simulink model "compressor"  (Simulink 7.4)
settings: Solver=ode45  StartTime=0.0  StopTime=10  MaxStep=0.01  RelTol=1e-3
values from neighbouring files (symbols this model uses):
  D = [-0.0083454 -0.0094965 0.16826 -0.032215 -0.61199 0.94175 -0.48522 0.10369]    [comp_coeffs.m]
  x_init_lin = [0.898 ... (first row only)    [MpcSetup.m]    (also in MpcSetup_linearized.m; compressor_setup.m; setup_compressor.m; test2.m = [0.899; 1.125; 0.1512; 440.7; 0])
libraries: dspsrcs4 x2, dspsnks4 x2
settings Model: Creator=chkajon  LastModifiedBy=chkajon

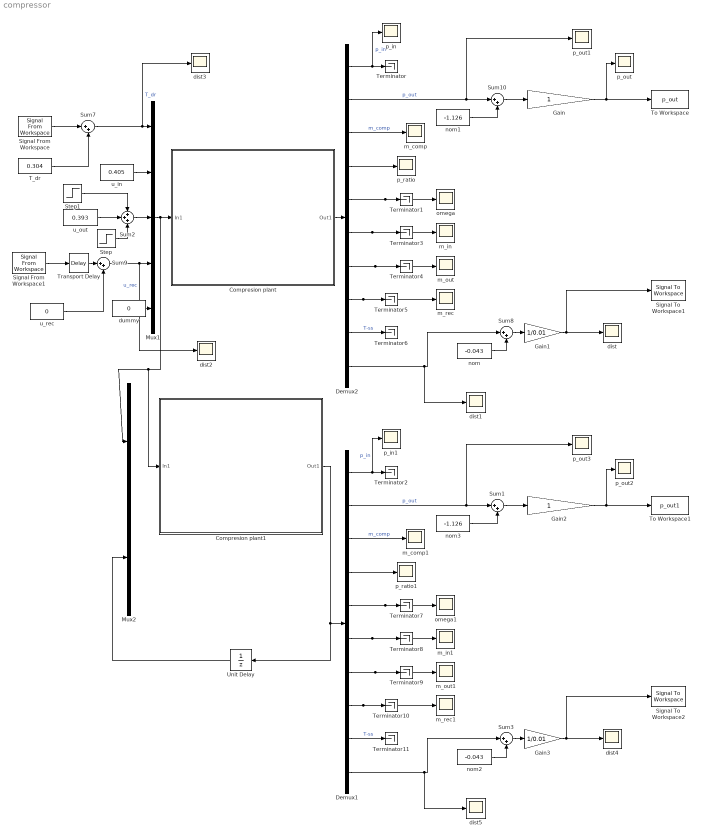
== system compressor ==
  Compresion plant : Subsystem
      mask Display: image(imread('comp_plant.jpg'))
  Compresion plant1 : Subsystem
      mask Display: image(imread('comp_plant.jpg'))
  Demux1 : Demux  Outputs=10
  Demux2 : Demux  Outputs=10
  Gain : Gain
  Gain1 : Gain  Gain=1/0.01
  Gain2 : Gain
  Gain3 : Gain  Gain=1/0.01
  Mux1 : Mux  Inputs=5
  Mux2 : Mux  Inputs=2
  Signal From Workspace : dspsrcs4/Signal From Workspace  SystemSampleTime=-1  X=Td  Ts=1  nsamps=1  OutputAfterFinalValue=Holding final value  ignoreOrWarnInputAndFrameLengths=off
  Signal From Workspace1 : dspsrcs4/Signal From Workspace  SystemSampleTime=-1  X=rec_open  Ts=1  nsamps=1  OutputAfterFinalValue=Holding final value  ignoreOrWarnInputAndFrameLengths=off
  Signal To Workspace1 : dspsnks4/Signal To Workspace  SystemSampleTime=-1  VariableName=SD  FrameMode=Concatenate frames (2-D array)
      settings: FixptAsFi=off
  Signal To Workspace2 : dspsnks4/Signal To Workspace  SystemSampleTime=-1  VariableName=SD1  FrameMode=Concatenate frames (2-D array)
      settings: FixptAsFi=off
  Step : Step  Time=50  After=-0.1  SampleTime=0
  Step1 : Step  Time=100  After=0  SampleTime=0
  Sum{1,3,7..10} (6 alike) : Sum  Inputs=|++
  Sum2 : Sum  Inputs=+++
  T_dr : Constant  Value=0.304
  Terminator{,1..11} (12 alike) : Terminator
  To Workspace : ToWorkspace  VariableName=p_out  SampleTime=-1  SaveFormat=Structure With Time
  To Workspace1 : ToWorkspace  VariableName=p_out1  SampleTime=-1  SaveFormat=Structure With Time
  Transport Delay : TransportDelay  DelayTime=1.0
  Unit Delay : UnitDelay  SampleTime=-1
  dist{,1..5} (6 alike) : Scope
      dist settings: YMin=-11  YMax=2
      dist1 settings: TimeRange=100  YMin=0.03  YMax=0.075
      dist2 settings: TimeRange=100  YMin=-0.25  YMax=1  SaveName=ScopeData3
      dist3 settings: TimeRange=100  YMin=-9  YMax=1  SaveName=ScopeData2
      dist4 settings: YMin=-11  YMax=2  SaveName=ScopeData11
      dist5 settings: TimeRange=100  YMin=0.03  YMax=0.075  SaveName=ScopeData12
  dummy : Constant  Value=0
  m_comp : Scope
      settings: TimeRange=100  YMin=0.5  YMax=0.825  SaveName=m_comp  DataFormat=Array
  m_comp1 : Scope
      settings: TimeRange=100  YMin=0.5  YMax=0.825  SaveName=m_comp1  DataFormat=Array
  m_in : Scope
      settings: TimeRange=100  YMin=100.8  YMax=100.975  SaveName=ScopeData4
  m_in1 : Scope
      settings: TimeRange=100  YMin=100.8  YMax=100.975  SaveName=ScopeData13
  m_out : Scope
      settings: TimeRange=100  YMin=100.8  YMax=100.975  SaveName=ScopeData5
  m_out1 : Scope
      settings: TimeRange=100  YMin=100.8  YMax=100.975  SaveName=ScopeData14
  m_rec : Scope
      settings: TimeRange=100  YMin=100.8  YMax=100.975  SaveName=ScopeData6
  m_rec1 : Scope
      settings: TimeRange=100  YMin=100.8  YMax=100.975  SaveName=ScopeData15
  nom : Constant  Value=-0.043
  nom1 : Constant  Value=-1.126
  nom2 : Constant  Value=-0.043
  nom3 : Constant  Value=-1.126
  omega : Scope
      settings: TimeRange=100  YMin=200  YMax=700  SaveName=ScopeData10
  omega1 : Scope
      settings: TimeRange=100  YMin=200  YMax=700  SaveName=ScopeData16
  p_in : Scope
      settings: TimeRange=100  YMin=0.895197  YMax=0.895225  SaveName=ScopeData9
  p_in1 : Scope
      settings: TimeRange=100  YMin=0.895197  YMax=0.895225  SaveName=ScopeData17
  p_out{,1..3} (4 alike) : Scope
      p_out settings: TimeRange=100  YMin=-2.5  YMax=40  SaveName=ScopeData7
      p_out1 settings: TimeRange=100  YMin=100.8  YMax=100.975  SaveName=ScopeData8
      p_out2 settings: TimeRange=100  YMin=-2.5  YMax=40  SaveName=ScopeData18
      p_out3 settings: TimeRange=100  YMin=100.8  YMax=100.975  SaveName=ScopeData19
  p_ratio : Scope
      settings: TimeRange=100  YMin=0.5  YMax=0.825  SaveName=p_ratio  DataFormat=Array
  p_ratio1 : Scope
      settings: TimeRange=100  YMin=0.5  YMax=0.825  SaveName=p_ratio1  DataFormat=Array
  u_in : Constant  Value=0.405
  u_out : Constant  Value=0.393
  u_rec : Constant  Value=0
  wires:
  Demux2/9 -> Terminator6/1  "T-ss"
  Sum2/1 -> Mux1/3
  Step/1 -> Sum2/3
  Transport Delay/1 -> Sum9/1
  dummy/1 -> Mux1/5
  Demux2/10 -> dist1/1, Sum8/1
  Gain1/1 -> dist/1, Signal To Workspace1/1
  Signal From Workspace/1 -> Sum7/1
  u_rec/1 -> Sum9/2
  T_dr/1 -> Sum7/2
  Gain/1 -> p_out/1, To Workspace/1
  nom1/1 -> Sum10/2
  Sum10/1 -> Gain/1
  Demux2/4 -> p_ratio/1
  Demux2/5 -> omega/1, Terminator1/1
  Demux2/1 -> p_in/1, Terminator/1  "p_in"
  Demux2/2 -> p_out1/1, Sum10/1  "p_out"
  Sum8/1 -> Gain1/1
  nom/1 -> Sum8/2
  Sum9/1 -> dist2/1, Mux1/4  "u_rec"
  Sum7/1 -> Mux1/1, dist3/1  "T_dr"
  Signal From Workspace1/1 -> Transport Delay/1
  u_out/1 -> Sum2/2
  Demux2/7 -> m_out/1, Terminator4/1
  Demux2/8 -> m_rec/1, Terminator5/1
  Demux2/6 -> m_in/1, Terminator3/1
  u_in/1 -> Mux1/2
  Demux2/3 -> m_comp/1  "m_comp"
  Mux1/1 -> Compresion plant/1(In1), Mux2/1, Compresion plant1/1(In1)
  Compresion plant/1(Out1) -> Demux2/1
  Step1/1 -> Sum2/1
  Demux1/9 -> Terminator11/1  "T-ss"
  Demux1/10 -> dist5/1, Sum3/1
  Gain3/1 -> dist4/1, Signal To Workspace2/1
  Gain2/1 -> p_out2/1, To Workspace1/1
  nom3/1 -> Sum1/2
  Sum1/1 -> Gain2/1
  Demux1/4 -> p_ratio1/1
  Demux1/5 -> omega1/1, Terminator7/1
  Demux1/1 -> p_in1/1, Terminator2/1  "p_in"
  Demux1/2 -> p_out3/1, Sum1/1  "p_out"
  Sum3/1 -> Gain3/1
  nom2/1 -> Sum3/2
  Demux1/7 -> m_out1/1, Terminator9/1
  Demux1/8 -> m_rec1/1, Terminator10/1
  Demux1/6 -> m_in1/1, Terminator8/1
  Demux1/3 -> m_comp1/1  "m_comp"
  Compresion plant1/1(Out1) -> Demux1/1, Unit Delay/1
  Unit Delay/1 -> Mux2/2

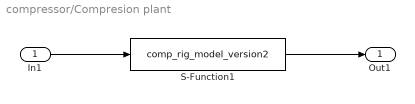
== system compressor/Compresion plant ==
  In1 : Inport
  S-Function1 : S-Function  FunctionName=comp_rig_model_version2  Parameters=[], x_init_lin  EnableBusSupport=off
  Out1 : Outport
  wires:
  In1/1 -> S-Function1/1
  S-Function1/1 -> Out1/1

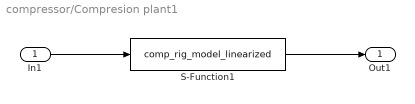
== system compressor/Compresion plant1 ==
  In1 : Inport
  S-Function1 : S-Function  FunctionName=comp_rig_model_linearized  Parameters=[], x_init_lin  EnableBusSupport=off
  Out1 : Outport
  wires:
  In1/1 -> S-Function1/1
  S-Function1/1 -> Out1/1
